simulink model "testbench_cp_fwd"  (R2015b)
settings: Solver=FixedStepAuto  StartTime=0.0  StopTime=inf  RelTol=1e-3
model workspace (MAT data in the model file):
  ratio = 0.1
libraries: legoev3lib x4
settings Model: SimulationMode=external  ExtModeTrigDuration=2  Creator=Shobhit  LastModifiedBy=Shobhit
settings SolverCC: PositivePriorityOrder=on
settings DataIOCC: LimitDataPoints=off
settings OptimizationCC: OptimizeModelRefInitCode=on  LifeSpan=1  MaxStackSize=64
settings DebuggingCC: ParameterPrecisionLossMsg=none  AllowSymbolicDim=on
settings HardwareCC: ProdBitPerPointer=32  ProdLargestAtomicInteger=Long  ProdWordSize=32  ProdHWDeviceType=ARM Compatible->ARM 9
settings ModelReferenceCC: PropagateSignalLabelsOutOfModel=on
settings RTWCC: SystemTargetFile=ert.tlc  TemplateMakefile=ert_default_tmf  Description=Embedded Coder  GenerateReport=on  Toolchain=Sourcery G++ Lite v2009q3  IncludeHyperlinkInReport=on  LaunchReport=on  GenerateTraceInfo=on  GenerateTraceReport=on  GenerateTraceReportSl=on  GenerateTraceReportSf=on  GenerateTraceReportEml=on
settings CodeAppCC: ForceParamTrailComments=on  IgnoreCustomStorageClasses=off  OperatorAnnotations=on  SimulinkDataObjDesc=on  SFDataObjDesc=on  MATLABFcnDesc=on  InsertBlockDesc=on  MATLABSourceComments=on
settings ERTTargetCC: SupportContinuousTime=on  SupportNonInlinedSFcns=on  SupportVariableSizeSignals=on  ConvertIfToSwitch=on  SuppressUnreachableDefaultCases=on

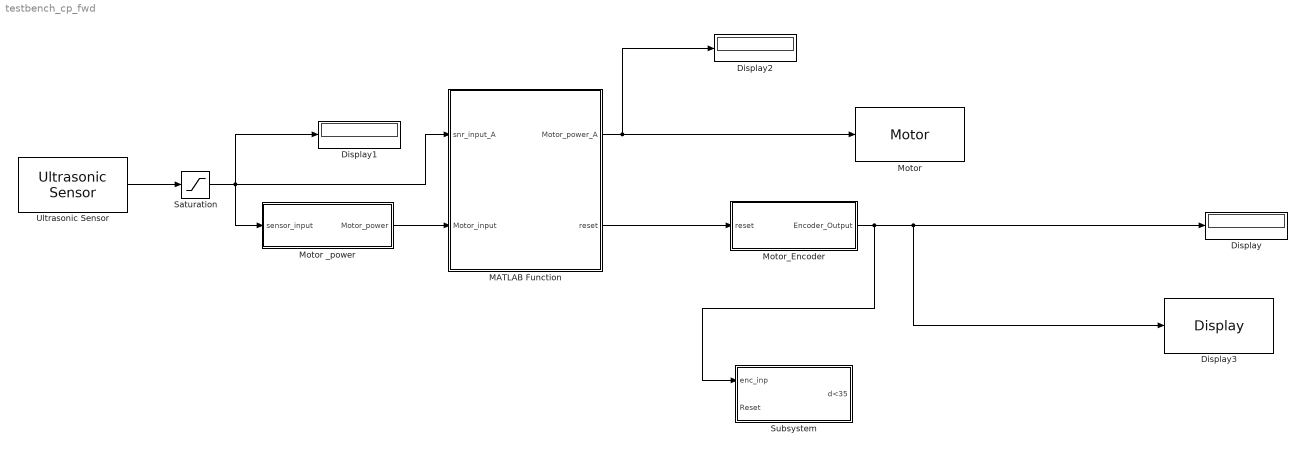
== system testbench_cp_fwd ==
  " Subsystem" : Subsystem  TreatAsAtomicUnit=on
  Display : Display
  Display1 : Display
  Display2 : Display
  Display3 : legoev3lib/Display  slcdLine=1  slcdFormat=Decimal
  MATLAB Function : MATLAB Function  TreatAsAtomicUnit=on
      settings: PermitHierarchicalResolution=ParametersOnly
  Motor : legoev3lib/Motor  sportNumber=A  sstopAction=Brake
  Motor _power : Subsystem
  Motor_Encoder : Subsystem
  Saturation : Saturate  UpperLimit=100  LowerLimit=3
  Ultrasonic Sensor : legoev3lib/Ultrasonic Sensor  PortNumber=1  sampleTime=0.1
  wires:
  Ultrasonic Sensor/1 -> Saturation/1
  MATLAB Function/1(Motor_power_A) -> Display2/1, Motor/1
  Saturation/1 -> Display1/1, MATLAB Function/1(snr_input_A), Motor _power/1(sensor_input)
  Motor _power/1("Motor_power ") -> MATLAB Function/2(Motor_input)
  Motor_Encoder/1(Encoder_Output) -> " Subsystem"/1(enc_inp), Display3/1, Display/1
  MATLAB Function/2(reset) -> Motor_Encoder/1(reset)

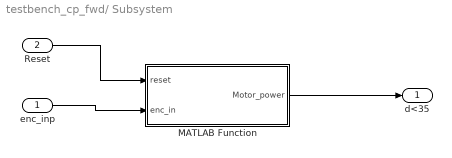
== system testbench_cp_fwd/ Subsystem ==
  enc_inp : Inport
  "Reset " : Inport  Port=2
  MATLAB Function : MATLAB Function  TreatAsAtomicUnit=on
      settings: PermitHierarchicalResolution=ParametersOnly
  d<35 : Outport
  wires:
  MATLAB Function/1(Motor_power) -> d<35/1
  enc_inp/1 -> MATLAB Function/2(enc_in)
  "Reset "/1 -> MATLAB Function/1(reset)

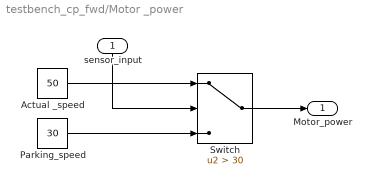
== system testbench_cp_fwd/Motor _power ==
  sensor_input : Inport
  Actual _speed : Constant  Value=50
  Parking_speed : Constant  Value=30
  Switch : Switch  Criteria=u2 > Threshold  Threshold=30
  "Motor_power " : Outport
  wires:
  Actual _speed/1 -> Switch/1
  Switch/1 -> "Motor_power "/1
  Parking_speed/1 -> Switch/3
  sensor_input/1 -> Switch/2

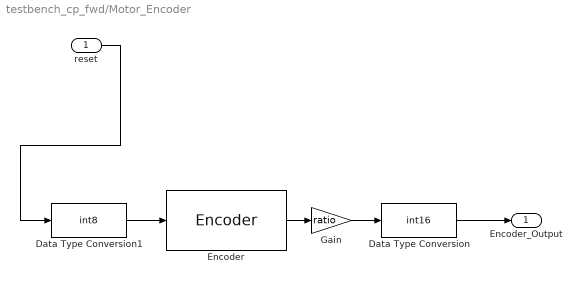
== system testbench_cp_fwd/Motor_Encoder ==
  reset : Inport
  Data Type Conversion : DataTypeConversion  OutDataTypeStr=int16  RndMeth=Round
  Data Type Conversion1 : DataTypeConversion  OutDataTypeStr=int8  RndMeth=Round
  Encoder : legoev3lib/Encoder  portNumber=A  opMode=Reset by external signal  sampleTime=0.1
  Gain : Gain  Gain=ratio
  Encoder_Output : Outport
  wires:
  reset/1 -> Data Type Conversion1/1
  Encoder/1 -> Gain/1
  Gain/1 -> Data Type Conversion/1
  Data Type Conversion/1 -> Encoder_Output/1
  Data Type Conversion1/1 -> Encoder/1

== matlab function testbench_cp_fwd/ Subsystem/MATLAB Function ==
  data: reset input; Motor_power output; enc_in input
function Motor_power = fcn(reset,enc_in)
%#codegen
if(reset==1)
    if(enc_in>=25)&&(enc_in<=35)
       Motor_power=0;
    else
       Motor_power= -50;
    end
else
    Motor_power=0;
end
end

== matlab function testbench_cp_fwd/MATLAB Function ==
  data: Motor_power_A output; reset output; snr_input_A input; Motor_input input
function [Motor_power_A,reset] = fcn(snr_input_A,Motor_input)
%#codegen
if(snr_input_A<=20)
    reset=1;
    Motor_power_A=Motor_input;
else
    Motor_power_A=Motor_input;
    reset=0;
end
end
